simulink model "WMRCTC"  (R2021a)
settings: Solver=FixedStepAuto  StartTime=0.0  StopTime=10  FixedStep=0.001  RelTol=1e-5
values from neighbouring files (symbols this model uses):
  d = 0.20    (= 0.2)    [WMR_Patameters.m]
  I = Ic + mc*d^2 + 2*mw*L^2    (= 0.420833333333)    [WMR_Patameters.m]
  Iw = 0.5*mw*R^2    (= 0.000125)    [WMR_Patameters.m]
  L = 0.25    [WMR_Patameters.m]
  m = mc + 2*mw    (= 5.2)    [WMR_Patameters.m]
  mc = 5.00    (= 5)    [WMR_Patameters.m]
  R = 0.05    [WMR_Patameters.m]
libraries: pid_lib x2
settings Model: Creator=power  LastModifiedBy=power

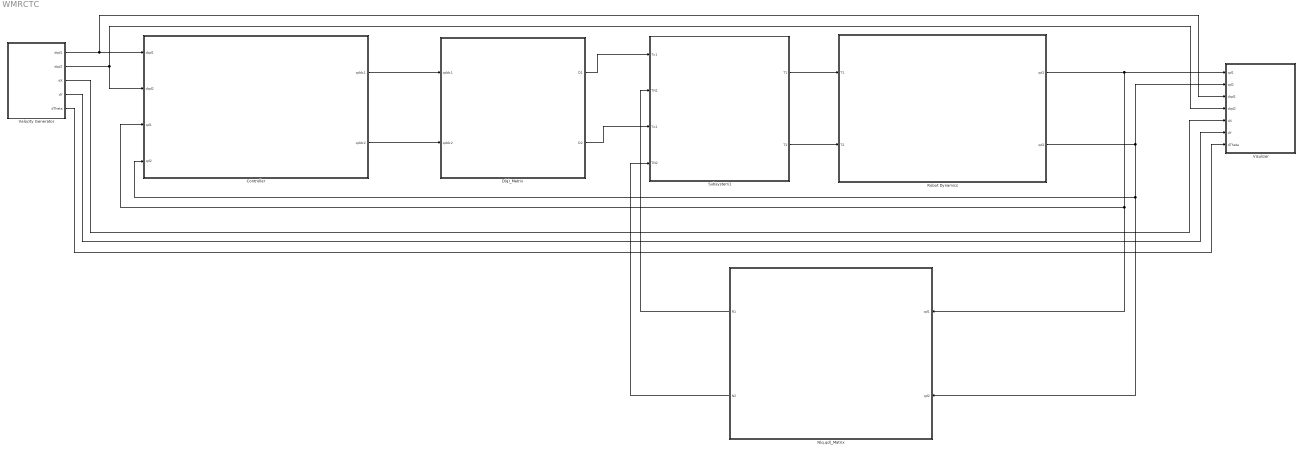
== system WMRCTC ==
  Controller : Subsystem
  D(q)_Matrix : Subsystem
  N(q,qd)_Matrix : Subsystem
  Robot Dynamics : Subsystem
  Subsystem1 : Subsystem
  Velocity Generator : Subsystem
  Visulizer : Subsystem
  wires:
  Velocity Generator/5(dTheta) -> Visulizer/7(dTheta)
  Velocity Generator/4(dY) -> Visulizer/6(dY)
  Velocity Generator/3(dX) -> Visulizer/5(dX)
  D(q)_Matrix/1(D1) -> Subsystem1/1(Tc1)
  D(q)_Matrix/2(D2) -> Subsystem1/3(Tc2)
  Subsystem1/2(T2) -> Robot Dynamics/2(T2)
  Velocity Generator/1(dqd1) -> Visulizer/3(dqd1), Controller/1(dqd1)
  Robot Dynamics/2(qd2) -> Visulizer/2(qd2), Controller/4(qd2), N(q,qd)_Matrix/2(qd2)
  Subsystem1/1(T1) -> Robot Dynamics/1(T1)
  Controller/1(qddc1) -> D(q)_Matrix/1(qddc1)
  N(q,qd)_Matrix/1(N1) -> Subsystem1/2(TN1)
  N(q,qd)_Matrix/2(N2) -> Subsystem1/4(TN2)
  Robot Dynamics/1(qd1) -> Visulizer/1(qd1), N(q,qd)_Matrix/1(qd1), Controller/3(qd1)
  Velocity Generator/2(dqd2) -> Controller/2(dqd2), Visulizer/4(dqd2)
  Controller/2(qddc2) -> D(q)_Matrix/2(qddc2)

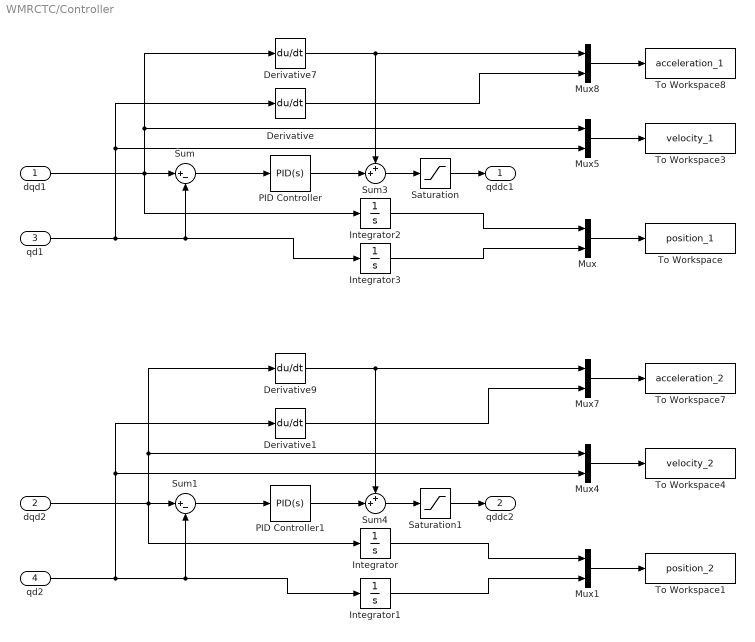
== system WMRCTC/Controller ==
  dqd1 : Inport
  dqd2 : Inport  Port=2
  qd1 : Inport  Port=3
  qd2 : Inport  Port=4
  Derivative{,1,7,9} (4 alike) : Derivative
  Integrator{,1..3} (4 alike) : Integrator
  Mux{,1,4..5,7..8} (6 alike) : Mux  Inputs=2
  PID Controller : pid_lib/PID Controller  Controller=PID  Form=Parallel  TimeDomain=Continuous-time  UseExternalTs=off  SampleTime=-1  IntegratorMethod=Forward Euler  FilterMethod=Forward Euler  ControllerParametersSource=internal  P=1.02763984168736  I=0.196569350266865  D=-0.216561164184195  UseFilter=on  N=1.72044274974478  TunerSelectOption=Transfer Function Based (PID Tuner App)  InitialConditionSource=internal  InitialConditionForIntegrator=0  InitialConditionForFilter=0  DifferentiatorICPrevScaledInput=0  ExternalReset=none  TrackingMode=off  Kt=1  LimitOutput=off  SatLimitsSource=internal  UpperSaturationLimit=inf  LowerSaturationLimit=-inf  LinearizeAsGain=on  AntiWindupMode=none  Kb=1  POutMin=[]  POutMax=[]  IOutMin=[]  IOutMax=[]  DOutMin=[]  DOutMax=[]  NOutMin=[]  NOutMax=[]  SumOutMin=[]  SumOutMax=[]  SaturationOutMin=[]  SaturationOutMax=[]  PParamMin=[]  PParamMax=[]  IParamMin=[]  IParamMax=[]  DParamMin=[]  DParamMax=[]  NParamMin=[]  NParamMax=[]  KbParamMin=[]  KbParamMax=[]  KtParamMin=[]  KtParamMax=[]  KbOutMin=[]  KbOutMax=[]  KtOutMin=[]  KtOutMax=[]  IntegratorOutMin=[]  IntegratorOutMax=[]  FilterOutMin=[]  FilterOutMax=[]  SumI1OutMin=[]  SumI1OutMax=[]  SumI2OutMin=[]  SumI2OutMax=[]  SumI3OutMin=[]  SumI3OutMax=[]  SumI4OutMin=[]  SumI4OutMax=[]  SumDOutMin=[]  SumDOutMax=[]  DifferentiatorOutMin=[]  DifferentiatorOutMax=[]  FilterDiffOutCoefMin=[]  FilterDiffOutCoefMax=[]  ReciprocalOutMin=[]  ReciprocalOutMax=[]  SumDenOutMin=[]  SumDenOutMax=[]  SumNumOutMin=[]  SumNumOutMax=[]  DivideOutMin=[]  DivideOutMax=[]  UdiffTsProdOutMin=[]  UdiffTsProdOutMax=[]  NTsProdOutMin=[]  NTsProdOutMax=[]  UintegralTsProdOutMin=[]  UintegralTsProdOutMax=[]  UngainTsProdOutMin=[]  UngainTsProdOutMax=[]  IntegratorContinuousStateAttributes=''  IntegratorStateMustResolveToSignalObject=off  IntegratorRTWStateStorageClass=Auto  FilterContinuousStateAttributes=''  FilterStateMustResolveToSignalObject=off  FilterRTWStateStorageClass=Auto  ParallelPVariant=InternalParameters  IdealPVariant=Disabled  IVariant=InternalParameters  DVariant=InternalParameters  IntegratorVariant=Continuous  SatVariant=Disabled  AWVariant=Passthrough  PCopyVariant=Disabled  TRVariant=Disabled  FdbkBlocksVariant=Forward  IdealPFdbkVariant=Disabled  SatFdbkVariant=Disabled  DerivativeFilterVariant=ContFilter  NVariant=InternalParameters  NCopyVariant=Disabled  FilterICVariant=InternalICsFilter  IntegratorICVariant=InternalICs  ExternalResetVariant=Disabled  TRSumVariant=Passthrough  SumFdbkVariant=Disabled  SumVariant=Sum_PID  TsampFilterVariant=InternalTs  TsampNgainVariant=Passthrough  TsampIntegralVariant=Passthrough  ExternalSaturationOutDataTypeStr=Inherit: Same as second input
  PID Controller1 : pid_lib/PID Controller  Controller=PID  Form=Parallel  TimeDomain=Continuous-time  UseExternalTs=off  SampleTime=-1  IntegratorMethod=Forward Euler  FilterMethod=Forward Euler  ControllerParametersSource=internal  P=1.02763984168736  I=0.196569350266865  D=-0.216561164184195  UseFilter=on  N=1.72044274974478  TunerSelectOption=Transfer Function Based (PID Tuner App)  InitialConditionSource=internal  InitialConditionForIntegrator=0  InitialConditionForFilter=0  DifferentiatorICPrevScaledInput=0  ExternalReset=none  TrackingMode=off  Kt=1  LimitOutput=off  SatLimitsSource=internal  UpperSaturationLimit=inf  LowerSaturationLimit=-inf  LinearizeAsGain=on  AntiWindupMode=none  Kb=1  POutMin=[]  POutMax=[]  IOutMin=[]  IOutMax=[]  DOutMin=[]  DOutMax=[]  NOutMin=[]  NOutMax=[]  SumOutMin=[]  SumOutMax=[]  SaturationOutMin=[]  SaturationOutMax=[]  PParamMin=[]  PParamMax=[]  IParamMin=[]  IParamMax=[]  DParamMin=[]  DParamMax=[]  NParamMin=[]  NParamMax=[]  KbParamMin=[]  KbParamMax=[]  KtParamMin=[]  KtParamMax=[]  KbOutMin=[]  KbOutMax=[]  KtOutMin=[]  KtOutMax=[]  IntegratorOutMin=[]  IntegratorOutMax=[]  FilterOutMin=[]  FilterOutMax=[]  SumI1OutMin=[]  SumI1OutMax=[]  SumI2OutMin=[]  SumI2OutMax=[]  SumI3OutMin=[]  SumI3OutMax=[]  SumI4OutMin=[]  SumI4OutMax=[]  SumDOutMin=[]  SumDOutMax=[]  DifferentiatorOutMin=[]  DifferentiatorOutMax=[]  FilterDiffOutCoefMin=[]  FilterDiffOutCoefMax=[]  ReciprocalOutMin=[]  ReciprocalOutMax=[]  SumDenOutMin=[]  SumDenOutMax=[]  SumNumOutMin=[]  SumNumOutMax=[]  DivideOutMin=[]  DivideOutMax=[]  UdiffTsProdOutMin=[]  UdiffTsProdOutMax=[]  NTsProdOutMin=[]  NTsProdOutMax=[]  UintegralTsProdOutMin=[]  UintegralTsProdOutMax=[]  UngainTsProdOutMin=[]  UngainTsProdOutMax=[]  IntegratorContinuousStateAttributes=''  IntegratorStateMustResolveToSignalObject=off  IntegratorRTWStateStorageClass=Auto  FilterContinuousStateAttributes=''  FilterStateMustResolveToSignalObject=off  FilterRTWStateStorageClass=Auto  ParallelPVariant=InternalParameters  IdealPVariant=Disabled  IVariant=InternalParameters  DVariant=InternalParameters  IntegratorVariant=Continuous  SatVariant=Disabled  AWVariant=Passthrough  PCopyVariant=Disabled  TRVariant=Disabled  FdbkBlocksVariant=Forward  IdealPFdbkVariant=Disabled  SatFdbkVariant=Disabled  DerivativeFilterVariant=ContFilter  NVariant=InternalParameters  NCopyVariant=Disabled  FilterICVariant=InternalICsFilter  IntegratorICVariant=InternalICs  ExternalResetVariant=Disabled  TRSumVariant=Passthrough  SumFdbkVariant=Disabled  SumVariant=Sum_PID  TsampFilterVariant=InternalTs  TsampNgainVariant=Passthrough  TsampIntegralVariant=Passthrough  ExternalSaturationOutDataTypeStr=Inherit: Same as second input
  Saturation : Saturate  UpperLimit=100  LowerLimit=-100
  Saturation1 : Saturate  UpperLimit=100  LowerLimit=-100
  Sum : Sum  Inputs=|+-
  Sum1 : Sum  Inputs=|+-
  Sum3 : Sum  Inputs=++|
  Sum4 : Sum  Inputs=++|
  To Workspace : ToWorkspace  VariableName=position_1  SaveFormat=Timeseries  SampleTime=-1
  To Workspace1 : ToWorkspace  VariableName=position_2  SaveFormat=Timeseries  SampleTime=-1
  To Workspace3 : ToWorkspace  VariableName=velocity_1  SaveFormat=Timeseries  SampleTime=-1
  To Workspace4 : ToWorkspace  VariableName=velocity_2  SaveFormat=Timeseries  SampleTime=-1
  To Workspace7 : ToWorkspace  VariableName=acceleration_2  SaveFormat=Timeseries  SampleTime=-1
  To Workspace8 : ToWorkspace  VariableName=acceleration_1  SaveFormat=Timeseries  SampleTime=-1
  qddc1 : Outport
  qddc2 : Outport  Port=2
  wires:
  Sum/1 -> PID Controller/1
  Sum1/1 -> PID Controller1/1
  Sum4/1 -> Saturation1/1
  PID Controller1/1 -> Sum4/2
  Sum3/1 -> Saturation/1
  PID Controller/1 -> Sum3/2
  dqd2/1 -> Integrator/1, Derivative9/1, Mux4/1, Sum1/1
  dqd1/1 -> Integrator2/1, Derivative7/1, Mux5/1, Sum/1
  Derivative/1 -> Mux8/2
  Derivative1/1 -> Mux7/2
  Mux/1 -> To Workspace/1
  Mux1/1 -> To Workspace1/1
  Mux4/1 -> To Workspace4/1
  Mux5/1 -> To Workspace3/1
  qd1/1 -> Mux5/2, Derivative/1, Integrator3/1, Sum/2
  qd2/1 -> Derivative1/1, Mux4/2, Integrator1/1, Sum1/2
  Mux7/1 -> To Workspace7/1
  Derivative9/1 -> Sum4/1, Mux7/1
  Mux8/1 -> To Workspace8/1
  Derivative7/1 -> Sum3/1, Mux8/1
  Integrator/1 -> Mux1/1
  Integrator1/1 -> Mux1/2
  Integrator2/1 -> Mux/1
  Integrator3/1 -> Mux/2
  Saturation/1 -> qddc1/1
  Saturation1/1 -> qddc2/1

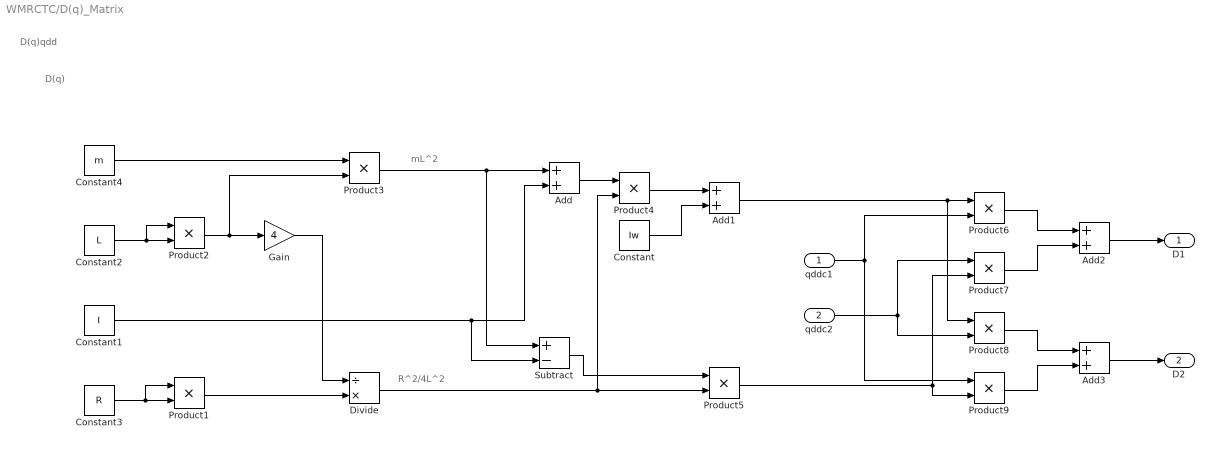
== system WMRCTC/D(q)_Matrix ==
  note: D(q)qdd
  note: D(q)
  note: R^2/4L^2
  note: mL^2
  qddc1 : Inport
  qddc2 : Inport  Port=2
  Add{,1..3} (4 alike) : Sum
  Constant : Constant  Value=Iw
  Constant1 : Constant  Value=I
  Constant2 : Constant  Value=L
  Constant3 : Constant  Value=R
  Constant4 : Constant  Value=m
  Divide : Product  Inputs=/*
  Gain : Gain  Gain=4
  Product{1..9} (9 alike) : Product
  Subtract : Sum  Inputs=+-
  D1 : Outport
  D2 : Outport  Port=2
  wires:
  Add2/1 -> D1/1
  Add3/1 -> D2/1
  qddc1/1 -> Product9/1, Product6/2
  qddc2/1 -> Product8/2, Product7/1
  Constant2/1 -> Product2/2, Product2/1
  Constant1/1 -> Subtract/2, Add/2
  Product3/1 -> Subtract/1, Add/1
  Constant3/1 -> Product1/1, Product1/2
  Constant4/1 -> Product3/1
  Product2/1 -> Gain/1, Product3/2
  Product1/1 -> Divide/2
  Gain/1 -> Divide/1
  Add/1 -> Product4/1
  Divide/1 -> Product5/2, Product4/2
  Product4/1 -> Add1/1
  Constant/1 -> Add1/2
  Subtract/1 -> Product5/1
  Add1/1 -> Product8/1, Product6/1
  Product5/1 -> Product9/2, Product7/2
  Product6/1 -> Add2/1
  Product7/1 -> Add2/2
  Product8/1 -> Add3/1
  Product9/1 -> Add3/2

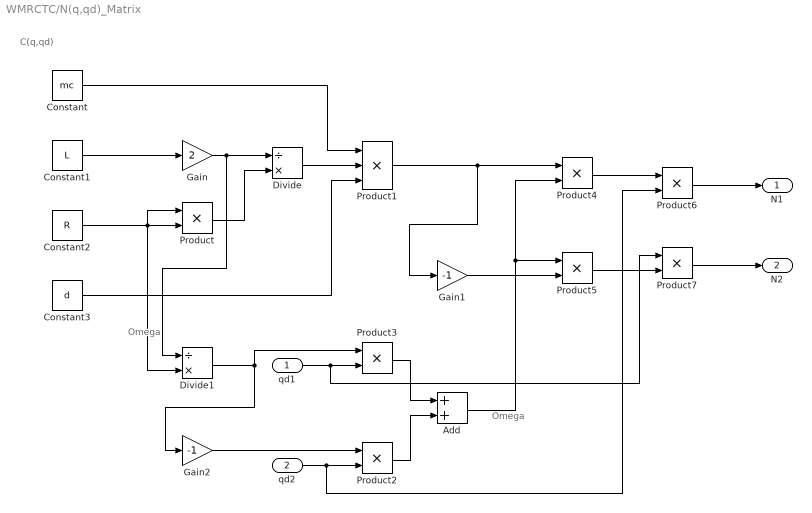
== system WMRCTC/N(q,qd)_Matrix ==
  note: C(q,qd)
  note: Omega
  note: Omega
  qd1 : Inport
  qd2 : Inport  Port=2
  Add : Sum
  Constant : Constant  Value=mc
  Constant1 : Constant  Value=L
  Constant2 : Constant  Value=R
  Constant3 : Constant  Value=d
  Divide : Product  Inputs=/*
  Divide1 : Product  Inputs=/*
  Gain : Gain  Gain=2
  Gain1 : Gain  Gain=-1
  Gain2 : Gain  Gain=-1
  Product{,2..7} (7 alike) : Product
  Product1 : Product  Inputs=3
  N1 : Outport
  N2 : Outport  Port=2
  wires:
  Product6/1 -> N1/1
  Product7/1 -> N2/1
  qd1/1 -> Product3/2, Product7/1
  Constant1/1 -> Gain/1
  Constant2/1 -> Divide1/2, Product/1, Product/2
  Gain/1 -> Divide1/1, Divide/1
  Product/1 -> Divide/2
  Divide/1 -> Product1/2
  Constant/1 -> Product1/1
  Constant3/1 -> Product1/3
  Product1/1 -> Product4/1, Gain1/1
  Divide1/1 -> Product3/1, Gain2/1
  qd2/1 -> Product6/2, Product2/2
  Gain2/1 -> Product2/1
  Product3/1 -> Add/1
  Product2/1 -> Add/2
  Gain1/1 -> Product5/2
  Add/1 -> Product4/2, Product5/1
  Product4/1 -> Product6/1
  Product5/1 -> Product7/2

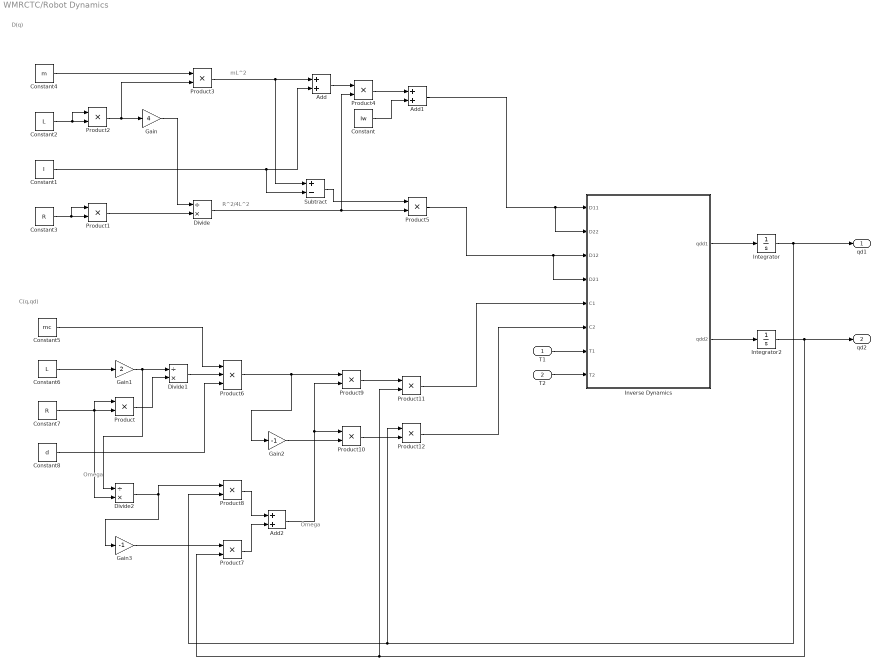
== system WMRCTC/Robot Dynamics ==
  note: D(q)
  note: R^2/4L^2
  note: mL^2
  note: C(q,qd)
  note: Omega
  note: Omega
  T1 : Inport
  T2 : Inport  Port=2
  Add : Sum
  Add1 : Sum
  Add2 : Sum
  Constant : Constant  Value=Iw
  Constant1 : Constant  Value=I
  Constant2 : Constant  Value=L
  Constant3 : Constant  Value=R
  Constant4 : Constant  Value=m
  Constant5 : Constant  Value=mc
  Constant6 : Constant  Value=L
  Constant7 : Constant  Value=R
  Constant8 : Constant  Value=d
  Divide : Product  Inputs=/*
  Divide1 : Product  Inputs=/*
  Divide2 : Product  Inputs=/*
  Gain : Gain  Gain=4
  Gain1 : Gain  Gain=2
  Gain2 : Gain  Gain=-1
  Gain3 : Gain  Gain=-1
  Integrator : Integrator
  Integrator2 : Integrator
  Inverse Dynamics : MATLAB Function  TreatAsAtomicUnit=on
  Product{,1..5,7..12} (12 alike) : Product
  Product6 : Product  Inputs=3
  Subtract : Sum  Inputs=+-
  qd1 : Outport
  qd2 : Outport  Port=2
  wires:
  Constant2/1 -> Product2/2, Product2/1
  Product4/1 -> Add1/1
  Product3/1 -> Subtract/1, Add/1
  Constant1/1 -> Subtract/2, Add/2
  Add/1 -> Product4/1
  Product1/1 -> Divide/2
  Divide/1 -> Product5/2, Product4/2
  Constant3/1 -> Product1/1, Product1/2
  Subtract/1 -> Product5/1
  Product2/1 -> Gain/1, Product3/2
  Constant/1 -> Add1/2
  Gain/1 -> Divide/1
  Constant4/1 -> Product3/1
  Constant8/1 -> Product6/3
  Gain1/1 -> Divide2/1, Divide1/1
  Product10/1 -> Product12/2
  Product7/1 -> Add2/2
  Product/1 -> Divide1/2
  Constant7/1 -> Divide2/2, Product/1, Product/2
  Integrator2/1 -> Product11/2, Product7/2, qd2/1
  Product6/1 -> Product9/1, Gain2/1
  Gain3/1 -> Product7/1
  Product8/1 -> Add2/1
  Divide1/1 -> Product6/2
  Constant5/1 -> Product6/1
  Integrator/1 -> Product12/1, Product8/2, qd1/1
  Divide2/1 -> Product8/1, Gain3/1
  Constant6/1 -> Gain1/1
  Product9/1 -> Product11/1
  Gain2/1 -> Product10/2
  Add2/1 -> Product9/2, Product10/1
  T2/1 -> Inverse Dynamics/8(T2)
  T1/1 -> Inverse Dynamics/7(T1)
  Product11/1 -> Inverse Dynamics/5(C1)
  Product12/1 -> Inverse Dynamics/6(C2)
  Add1/1 -> Inverse Dynamics/2(D22), Inverse Dynamics/1(D11)
  Product5/1 -> Inverse Dynamics/4(D21), Inverse Dynamics/3(D12)
  Inverse Dynamics/1(qdd1) -> Integrator/1
  Inverse Dynamics/2(qdd2) -> Integrator2/1

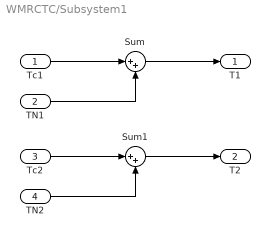
== system WMRCTC/Subsystem1 ==
  Tc1 : Inport
  TN1 : Inport  Port=2
  Tc2 : Inport  Port=3
  TN2 : Inport  Port=4
  Sum : Sum  Inputs=|++
  Sum1 : Sum  Inputs=|++
  T1 : Outport
  T2 : Outport  Port=2
  wires:
  Sum/1 -> T1/1
  Tc1/1 -> Sum/1
  TN1/1 -> Sum/2
  TN2/1 -> Sum1/2
  Tc2/1 -> Sum1/1
  Sum1/1 -> T2/1

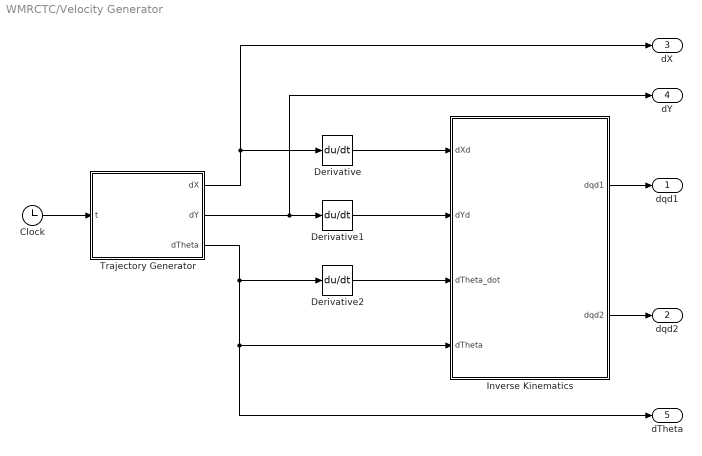
== system WMRCTC/Velocity Generator ==
  Clock : Clock
  Derivative : Derivative
  Derivative1 : Derivative
  Derivative2 : Derivative
  Inverse Kinematics : MATLAB Function  TreatAsAtomicUnit=on
  Trajectory Generator : MATLAB Function  TreatAsAtomicUnit=on
  dqd1 : Outport
  dqd2 : Outport  Port=2
  dX : Outport  Port=3
  dY : Outport  Port=4
  dTheta : Outport  Port=5
  wires:
  Clock/1 -> Trajectory Generator/1(t)
  Derivative/1 -> Inverse Kinematics/1(dXd)
  Derivative1/1 -> Inverse Kinematics/2(dYd)
  Derivative2/1 -> Inverse Kinematics/3(dTheta_dot)
  Trajectory Generator/1(dX) -> dX/1, Derivative/1
  Trajectory Generator/2(dY) -> dY/1, Derivative1/1
  Trajectory Generator/3(dTheta) -> dTheta/1, Inverse Kinematics/4(dTheta), Derivative2/1
  Inverse Kinematics/1(dqd1) -> dqd1/1
  Inverse Kinematics/2(dqd2) -> dqd2/1

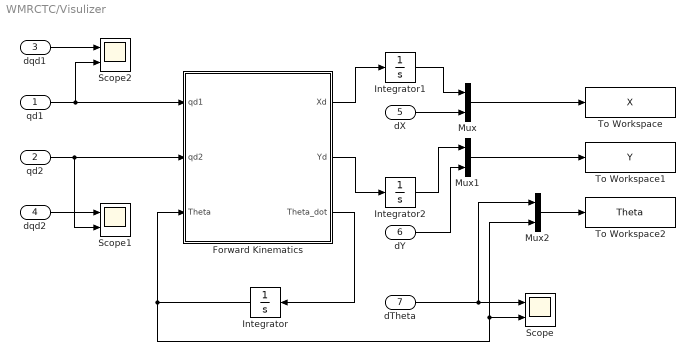
== system WMRCTC/Visulizer ==
  qd1 : Inport
  qd2 : Inport  Port=2
  dqd1 : Inport  Port=3
  dqd2 : Inport  Port=4
  dX : Inport  Port=5
  dY : Inport  Port=6
  dTheta : Inport  Port=7
  Forward Kinematics : MATLAB Function  TreatAsAtomicUnit=on
  Integrator : Integrator  InitialCondition=-pi/2
  Integrator1 : Integrator  InitialCondition=3
  Integrator2 : Integrator
  Mux : Mux  Inputs=2
  Mux1 : Mux  Inputs=2
  Mux2 : Mux  Inputs=2
  Scope : Scope  NumInputPorts=2
  Scope1 : Scope  NumInputPorts=2
  Scope2 : Scope  NumInputPorts=2
  To Workspace : ToWorkspace  VariableName=X  SaveFormat=Timeseries  SampleTime=-1
      settings: Save2DSignal=2-D array (concatenate along first dimension)
  To Workspace1 : ToWorkspace  VariableName=Y  SaveFormat=Timeseries  SampleTime=-1
      settings: Save2DSignal=2-D array (concatenate along first dimension)
  To Workspace2 : ToWorkspace  VariableName=Theta  SaveFormat=Timeseries  SampleTime=-1
      settings: Save2DSignal=2-D array (concatenate along first dimension)
  wires:
  Integrator/1 -> Mux2/2, Scope/2, Forward Kinematics/3(Theta)
  Forward Kinematics/3(Theta_dot) -> Integrator/1
  Forward Kinematics/2(Yd) -> Integrator2/1
  Forward Kinematics/1(Xd) -> Integrator1/1
  qd1/1 -> Scope2/2, Forward Kinematics/1(qd1)
  qd2/1 -> Scope1/2, Forward Kinematics/2(qd2)
  dqd1/1 -> Scope2/1
  dqd2/1 -> Scope1/1
  dTheta/1 -> Mux2/1, Scope/1
  Integrator2/1 -> Mux1/1
  Integrator1/1 -> Mux/1
  Mux/1 -> To Workspace/1
  Mux1/1 -> To Workspace1/1
  dX/1 -> Mux/2
  dY/1 -> Mux1/2
  Mux2/1 -> To Workspace2/1

== matlab function WMRCTC/Visulizer/Forward Kinematics ==
  data: qd1 input; Xd output; qd2 input; Theta input; Yd output; Theta_dot output; R parameter; L parameter
function [Xd,Yd,Theta_dot] = for_kin(qd1,qd2,Theta,R, L)
    
    %FOR_KIN Solve inverse kinematics
    %   FOR_KIN(xd,yd,td,t) takes three input arguments representing the
    %   robot wheels velocities. It also takes the robot orientation t,
    %   solve forward kinematics for these values, and then return the
    %   robot velocities wrt to the inertial frame.
    
    forward_kinematics_matrix = [R/2*cos(Theta),R/2*cos(Theta);
                                 R/2*sin(Theta),R/2*sin(Theta);
                                 R/(2*L)       ,-R/(2*L)];
    wheels_velocities_matrix = [qd1;qd2];
    
    inertial_frame_velocities = forward_kinematics_matrix*wheels_velocities_matrix;
    
    Xd = inertial_frame_velocities(1);
    Yd = inertial_frame_velocities(2);
    Theta_dot = inertial_frame_velocities(3);
end

== matlab function WMRCTC/Robot Dynamics/Inverse Dynamics ==
  data: D11 input; D22 input; qdd1 output; D12 input; D21 input; C1 input; C2 input; T1 input; T2 input; qdd2 output
function [qdd1,qdd2] = inverse_dynamics(D11,D22,D12,D21,C1,C2,T1,T2)

    %T_Matrix
    T = [T1;
         T2];
    
    %C_Matrix
    C = [C1;
         C2];
    
    %D_Matrix
    D = [D11,D12;
         D21,D22];
    
    %qdd_Matrix
    qdd = D \ (T - C);
    
    %Output
    qdd1 = qdd(1);
    qdd2 = qdd(2);
    
end

== matlab function WMRCTC/Velocity Generator/Inverse Kinematics ==
  data: dXd input; dqd1 output; dYd input; dTheta_dot input; dTheta input; dqd2 output; R parameter; L parameter
function [dqd1,dqd2] = inv_kin(dXd,dYd,dTheta_dot,dTheta,R,L)
    
    %INV_KIN Solve inverse kinematics
    %   INV_KIN(xd,yd,td,t) takes four input arguments representing the
    %   robot velocities wrt the inertial frame, xd, yd, and td. It also
    %   takes the robot orientation t, solve inverse kinematics for these
    %   values, and then return the robot wheels velocities.
    
    forward_kinematics_matrix = [R/2*cos(dTheta),R/2*cos(dTheta);
                                 R/2*sin(dTheta),R/2*sin(dTheta);
                                 R/(2*L)       ,-R/(2*L)];
    inertial_frame_velocities = [dXd;dYd;dTheta_dot];
    
    wheels_velocities_matrix = forward_kinematics_matrix\inertial_frame_velocities;
    
    dqd1 =  wheels_velocities_matrix(1);
    dqd2 =  wheels_velocities_matrix(2);
end

== matlab function WMRCTC/Velocity Generator/Trajectory Generator ==
  data: dX output; t input; dY output; dTheta output
function [dX,dY,dTheta] = traject_gen(t)
    
    %TRAJECT_GEN Trajectory Generator
    %   TRAJECT_GEN(t) takes time samples as input argument and return x
    %   position, y position, and the orientation for the infinity path.
    
    dX = 3*cos(t/10)/(1 + sin(t/10)^2);              % X-Position
    dY = 4*sin(t/10)*cos(t/10)/(1 + sin(t/10)^2);    % Y-Position
    % Orientation
    dTheta = atan(-(12*sin(t/10)^2 - 4)/(3*sin(t/10)*(sin(t/10)^2 - 3))) - ~(t < 10*pi)*pi;

end
